simulink model "RLC_Schwingkreis_s"  (R2019b)
settings: Solver=VariableStepAuto  StartTime=0.0  StopTime=0.1  RelTol=1e-6
values from neighbouring files (symbols this model uses):
  C = 2e-6    (= 2e-06)    [RLC_Schwingkreis_m.m]
  L = 0.24    [RLC_Schwingkreis_m.m]
  R = 100    [RLC_Schwingkreis_m.m]
  U_e = 5    [RLC_Schwingkreis_m.m]
settings Model: Creator=Arnulf  LastModifiedBy=dimad
settings DataIOCC: SaveFormat=Array

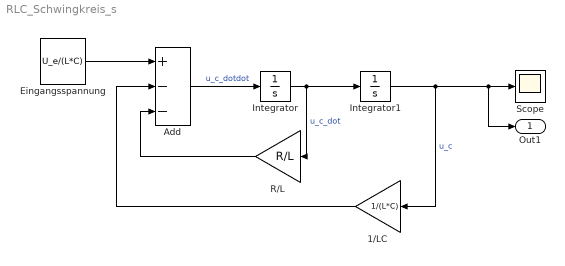
== system RLC_Schwingkreis_s ==
  1/LC : Gain  Gain=1/(L*C)
  Add : Sum  Inputs=+--
  Eingangsspannung : Constant  Value=U_e/(L*C)
  Integrator : Integrator
  Integrator1 : Integrator
  R/L : Gain  Gain=R/L
  Scope : Scope
  Out1 : Outport
  wires:
  Integrator/1 -> R/L/1, Integrator1/1  "u_c_dot"
  Add/1 -> Integrator/1  "u_c_dotdot"
  Integrator1/1 -> Out1/1, Scope/1, 1/LC/1  "u_c"
  Eingangsspannung/1 -> Add/1
  R/L/1 -> Add/3
  1/LC/1 -> Add/2
